simulink model "Prob9"  (R2020b)
settings: Solver=VariableStepAuto  StartTime=0.0  StopTime=10.0  RelTol=1e-3
model workspace (MAT data in the model file):
  J = Simulink.Parameter
  J.Value = 0.01
  J.DataType = 'auto'
  J.Dimensions = [1 1]
  K = Simulink.Parameter
  K.Value = 0.01
  K.DataType = 'auto'
  K.Dimensions = [1 1]
  L = Simulink.Parameter
  L.Value = 0.5
  L.DataType = 'auto'
  L.Dimensions = [1 1]
  R = Simulink.Parameter
  R.Value = 1
  R.DataType = 'auto'
  R.Dimensions = [1 1]
  b = Simulink.Parameter
  b.Value = 0.1
  b.DataType = 'auto'
  b.Dimensions = [1 1]
settings Model: Creator=shoun  LastModifiedBy=shoun

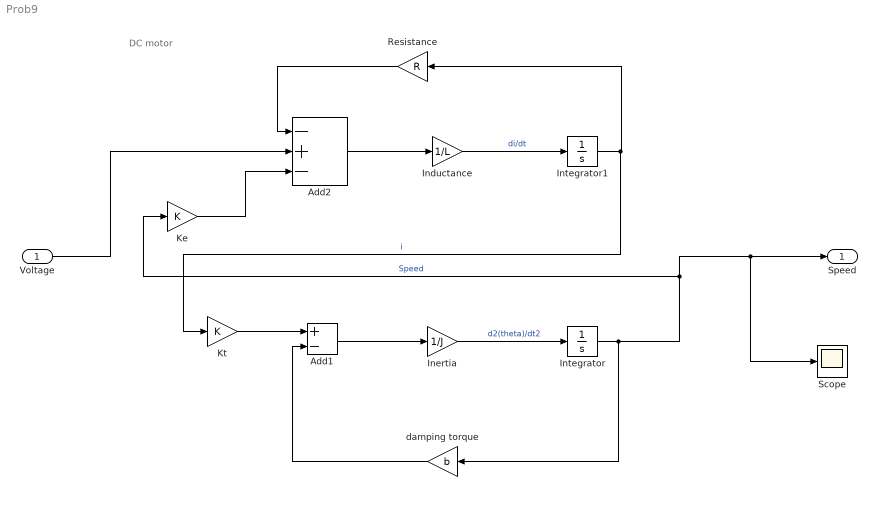
== system Prob9 ==
  note: DC motor
  Voltage : Inport
  Add1 : Sum  Inputs=+-
  Add2 : Sum  Inputs=-+-
  Inductance : Gain  Gain=1/L
  Inertia : Gain  Gain=1/J
  Integrator : Integrator
  Integrator1 : Integrator
  Ke : Gain  Gain=K
  Kt : Gain  Gain=K
  Resistance : Gain  Gain=R
  Scope : Scope
  damping torque : Gain  Gain=b
  Speed : Outport
  wires:
  Kt/1 -> Add1/1
  Add1/1 -> Inertia/1
  Inertia/1 -> Integrator/1  "d2(theta)/dt2"
  Integrator/1 -> damping torque/1, Ke/1, Scope/1, Speed/1  "Speed"
  Ke/1 -> Add2/3
  Voltage/1 -> Add2/2
  Add2/1 -> Inductance/1
  Inductance/1 -> Integrator1/1  "di/dt"
  Resistance/1 -> Add2/1
  Integrator1/1 -> Kt/1, Resistance/1  "i"
  damping torque/1 -> Add1/2
